simulink model "PROBLEM_2_SUSPENSION_SYSTEM"  (R2020b)
settings: Solver=VariableStepAuto  StartTime=0.0  StopTime=10.0  RelTol=1e-3
model workspace (MAT data in the model file):
  a = [-1.435  -0.2225  -0.0042  -0.0003; 1  0  0  0; 0  1  0  0; 0  0  1  0]
  b = [1; 0; 0; 0]
  c = [0 0 0.0042 0.0003]
  d = 0
  den = [1000 1435 222.5 4.2 0.3]
  num = [4.2 0.3]
  out = Simulink.SimulationOutput
  out.Data.logsout = Simulink.SimulationData.Dataset
  out.Data.logsout.any.Name = 'logsout'
  out.Data.logsout.any.Version = 3
  out.Data.logsout.any.Storage = Simulink.SimulationData.Storage.RamDatasetStorage
  out.Data.logsout.any.Storage.any.Version = 2
  out.Data.logsout.any.Storage.any.Elements{1} = Simulink.SimulationData.Signal
  out.Data.logsout.any.Storage.any.Elements{1}.PortType = 'outport'
  out.Data.logsout.any.Storage.any.Elements{1}.Version = 1
  out.Data.logsout.any.Storage.any.Elements{1}.BlockPath = Simulink.SimulationData.BlockPath
  out.Data.logsout.any.Storage.any.Elements{1}.BlockPath.path = {'PROBLEM_2_SUSPENSION_SYSTEM/Randum Signal Generator'}
  out.Data.logsout.any.Storage.any.Elements{1}.Values = timeseries
  out.Data.logsout.any.Storage.any.Elements{1}.Values.DataInfo = tsdata.datametadata
  out.Data.logsout.any.Storage.any.Elements{1}.Values.DataInfo.Interpolation = tsdata.interpolation
  out.Data.logsout.any.Storage.any.Elements{1}.Values.DataInfo.Interpolation.Fhandle : function handle (value not decoded)
  out.Data.logsout.any.Storage.any.Elements{1}.Values.DataInfo.Interpolation.Name = 'zoh'
  out.Data.logsout.any.Storage.any.Elements{1}.Values.TimeInfo = tsdata.timemetadata
  out.Data.logsout.any.Storage.any.Elements{1}.Values.TimeInfo.Length = 55
  out.Data.logsout.any.Storage.any.Elements{1}.Values.TimeInfo.DuplicateTimes = 0
  out.Data.logsout.any.Storage.any.Elements{1}.Values.TimeInfo.Time_ = [0; 0.000357511978234; 0.0021450718694; 0.0110828713253; 0.0557718686045; 0.255771868605; 0.453364954523; 0.653364954523; 0.853364954523; 1.05336495452; 1.25336495452; 1.45336495452; 1.65336495452; 1.85336495452; 2.05336495452; 2.25336495452; 2.45336495452; 2.65336495452; 2.85336495452; 3.05336495452; 3.25336495452; 3.45336495452; 3.65336495452; 3.85336495452; 4.05336495452; 4.25336495452; 4.45336495452; 4.65336495452; 4.85336495452; 5.05336495452; 5.25336495452; 5.45336495452; 5.65336495452; 5.85336495452; 6.05336495452; 6.25336495452; 6.45336495452; 6.65336495452; 6.85336495452; 7.05336495452; 7.25336495452; 7.45336495452; 7.65336495452; 7.85336495452; 8.05336495452; 8.25336495452; 8.45336495452; 8.65336495452; 8.85336495452; 9.05336495452; 9.25336495452; 9.45336495452; 9.65336495452; 9.85336495452; 10]
  out.Data.logsout.any.Storage.any.Elements{1}.Values.TimeInfo.Initialized = 1
  out.Data.logsout.any.Storage.any.Elements{1}.Values.QualityInfo = tsdata.qualmetadata
  out.Data.logsout.any.Storage.any.Elements{1}.Values.Data_ = [-0.562081627344; -0.905910767571; 0.357729433737; 0.358592811673; 0.869385791882; -0.23299584502; 0.0388327441359; 0.661930692225; -0.930855778945; -0.893076729911; 0.0594003866703; 0.342298768154; -0.984603627578; -0.23316869849; -0.866315524963; -0.165028051084; 0.373545424721; 0.177953285714; 0.860872989456; 0.692333781017; 0.0538575551723; -0.816070218485; 0.307837924598; -0.168001286298; 0.402381188889; 0.820641660979; 0.524396079371; -0.475094012672; -0.905070972585; 0.472163769171; -0.34353154774; 0.265277135775; 0.512820971903; 0.982074771068; -0.269322658549; -0.505922228799; 0.965100572428; 0.445320801551; 0.506711669968; 0.303037149507; -0.854628234103; 0.263269436203; 0.769414257151; -0.454580066472; -0.127177188698; 0.532989555752; -0.0445364699906; -0.524451132642; -0.450186319393; -0.281470041387; -0.666985599169; -0.0269652339755; 0.795312573107; 0.818416203288; -0.878871344905]
  out.Data.logsout.any.Storage.any.Elements{2} = Simulink.SimulationData.Signal
  out.Data.logsout.any.Storage.any.Elements{2}.PortType = 'outport'
  out.Data.logsout.any.Storage.any.Elements{2}.Version = 1
  out.Data.logsout.any.Storage.any.Elements{2}.BlockPath = Simulink.SimulationData.BlockPath
  out.Data.logsout.any.Storage.any.Elements{2}.BlockPath.path = {'PROBLEM_2_SUSPENSION_SYSTEM/transfer Fcn'}
  out.Data.logsout.any.Storage.any.Elements{2}.Values = timeseries
  out.Data.logsout.any.Storage.any.Elements{2}.Values.DataInfo = tsdata.datametadata
  out.Data.logsout.any.Storage.any.Elements{2}.Values.DataInfo.Interpolation = tsdata.interpolation
  out.Data.logsout.any.Storage.any.Elements{2}.Values.DataInfo.Interpolation.Fhandle : function handle (value not decoded)
  out.Data.logsout.any.Storage.any.Elements{2}.Values.DataInfo.Interpolation.Name = 'linear'
  out.Data.logsout.any.Storage.any.Elements{2}.Values.TimeInfo = tsdata.timemetadata
  out.Data.logsout.any.Storage.any.Elements{2}.Values.TimeInfo.Length = 55
  out.Data.logsout.any.Storage.any.Elements{2}.Values.TimeInfo.DuplicateTimes = 0
  out.Data.logsout.any.Storage.any.Elements{2}.Values.TimeInfo.Time_ = [0; 0.000357511978234; 0.0021450718694; 0.0110828713253; 0.0557718686045; 0.255771868605; 0.453364954523; 0.653364954523; 0.853364954523; 1.05336495452; 1.25336495452; 1.45336495452; 1.65336495452; 1.85336495452; 2.05336495452; 2.25336495452; 2.45336495452; 2.65336495452; 2.85336495452; 3.05336495452; 3.25336495452; 3.45336495452; 3.65336495452; 3.85336495452; 4.05336495452; 4.25336495452; 4.45336495452; 4.65336495452; 4.85336495452; 5.05336495452; 5.25336495452; 5.45336495452; 5.65336495452; 5.85336495452; 6.05336495452; 6.25336495452; 6.45336495452; 6.65336495452; 6.85336495452; 7.05336495452; 7.25336495452; 7.45336495452; 7.65336495452; 7.85336495452; 8.05336495452; 8.25336495452; 8.45336495452; 8.65336495452; 8.85336495452; 9.05336495452; 9.25336495452; 9.45336495452; 9.65336495452; 9.85336495452; 10]
  out.Data.logsout.any.Storage.any.Elements{2}.Values.TimeInfo.Initialized = 1
  out.Data.logsout.any.Storage.any.Elements{2}.Values.QualityInfo = tsdata.qualmetadata
  out.Data.logsout.any.Storage.any.Elements{2}.Values.Data_ = [0; -1.79769617365e-14; -5.2545676181e-12; -1.99823284744e-10; 2.68404498816e-08; 6.21540832091e-06; 3.33796218492e-05; 7.66765863418e-05; 0.000135083595736; 0.000213011794581; 0.000285578520613; 0.000332316235162; 0.000358070547876; 0.000369568723865; 0.000351228771915; 0.000296660223416; 0.000195857608614; 5.50687074212e-05; -0.000108048435281; -0.000277752458139; -0.000430433823258; -0.000551722669519; -0.000648653887148; -0.000740766542261; -0.000827409016616; -0.000909310861356; -0.000975860507589; -0.00100979959918; -0.00100725901542; -0.000988637627288; -0.000975312475436; -0.000962789878736; -0.000954142409177; -0.000942195435816; -0.000911411736333; -0.000846273078161; -0.000758722946634; -0.000660598580283; -0.000535940247566; -0.000375849169482; -0.000175939543201; 5.71877376748e-05; 0.000300614028672; 0.000556114151792; 0.000833607921404; 0.00112060861772; 0.00141185503937; 0.00171473594978; 0.00202402370516; 0.00232406756258; 0.00260314669473; 0.00285406285464; 0.00306803595231; 0.00325363092994; 0.00338660884517]
  out.Data.tout = [0; 0.000357511978234; 0.0021450718694; 0.0110828713253; 0.0557718686045; 0.255771868605; 0.453364954523; 0.653364954523; 0.853364954523; 1.05336495452; 1.25336495452; 1.45336495452; 1.65336495452; 1.85336495452; 2.05336495452; 2.25336495452; 2.45336495452; 2.65336495452; 2.85336495452; 3.05336495452; 3.25336495452; 3.45336495452; 3.65336495452; 3.85336495452; 4.05336495452; 4.25336495452; 4.45336495452; 4.65336495452; 4.85336495452; 5.05336495452; 5.25336495452; 5.45336495452; 5.65336495452; 5.85336495452; 6.05336495452; 6.25336495452; 6.45336495452; 6.65336495452; 6.85336495452; 7.05336495452; 7.25336495452; 7.45336495452; 7.65336495452; 7.85336495452; 8.05336495452; 8.25336495452; 8.45336495452; 8.65336495452; 8.85336495452; 9.05336495452; 9.25336495452; 9.45336495452; 9.65336495452; 9.85336495452; 10]
  out.Metadata = Simulink.SimulationMetadata
  out.Metadata.ModelInfo.ModelName = 'PROBLEM_2_SUSPENSION_SYSTEM'
  out.Metadata.ModelInfo.ModelVersion = '1.3'
  out.Metadata.ModelInfo.ModelFilePath = 'D:\KPIT\PROBLEM_2\Simulink Model\PROBLEM_2_SUSPENSION_SYSTEM.slx'
  out.Metadata.ModelInfo.UserID = 'intel'
  out.Metadata.ModelInfo.MachineName = 'DESKTOP-HTPAP2M'
  out.Metadata.ModelInfo.Platform = 'PCWIN64'
  out.Metadata.ModelInfo.ModelStructuralChecksum = [2786829521; 1170271611; 2990410611; 2656339131]
  out.Metadata.ModelInfo.SimulationMode = 'normal'
  out.Metadata.ModelInfo.StartTime = 0
  out.Metadata.ModelInfo.StopTime = 10
  out.Metadata.ModelInfo.SolverInfo.Type = 'Variable-Step'
  out.Metadata.ModelInfo.SolverInfo.Solver = 'ode45'
  out.Metadata.ModelInfo.SolverInfo.MaxStepSize = 0.2
  out.Metadata.ModelInfo.SimulinkVersion.Name = 'Simulink'
  out.Metadata.ModelInfo.SimulinkVersion.Version = '10.2'
  out.Metadata.ModelInfo.SimulinkVersion.Release = '(R2020b)'
  out.Metadata.ModelInfo.SimulinkVersion.Date = '29-Jul-2020'
  out.Metadata.ModelInfo.LoggingInfo.LoggingToFile = 'off'
  out.Metadata.TimingInfo.WallClockTimestampStart = '2020-12-04 22:57:30'
  out.Metadata.TimingInfo.WallClockTimestampStop = '2020-12-04 22:57:32'
  out.Metadata.TimingInfo.InitializationElapsedWallTime = 1.1649333
  out.Metadata.TimingInfo.ExecutionElapsedWallTime = 0.3698049
  out.Metadata.TimingInfo.TerminationElapsedWallTime = 0.268201
  out.Metadata.TimingInfo.TotalElapsedWallTime = 1.8029392
  out.Metadata.TimingInfo.ProfilerData = 'Profiler is not enabled'
  out.Metadata.ExecutionInfo.StopEvent = 'ReachedStopTime'
  out.Metadata.ExecutionInfo.StopEventSource = []
  out.Metadata.ExecutionInfo.StopEventDescription = 'Reached stop time of 10'
  out.Metadata.ExecutionInfo.ErrorDiagnostic = []
  out.Metadata.ExecutionInfo.WarningDiagnostics.Diagnostic = MSLDiagnostic
  out.Metadata.ExecutionInfo.WarningDiagnostics.Diagnostic.identifier = 'Simulink:blocks:SiggenRandomWaveObsolete'
  out.Metadata.ExecutionInfo.WarningDiagnostics.Diagnostic.message = 'The "random" waveform selection of ''<a href="matlab:open_and_hilite_hyperlink (''PROBLEM_2_SUSPENSION_SYSTEM/Randum Signal Generator'',''error'')">PROBLEM_2_SUSPENSION_SYSTEM/Randum Signal Generator</a>'' is provided for backwards compatibility. It will be removed in a future version and should be replaced with the appropriate random number generator'
  out.Metadata.ExecutionInfo.WarningDiagnostics.Diagnostic.paths = {'PROBLEM_2_SUSPENSION_SYSTEM/Randum Signal Generator'}
  out.Metadata.ExecutionInfo.WarningDiagnostics.Diagnostic.arguments = {'PROBLEM_2_SUSPENSION_SYSTEM/Randum Signal Generator'}
  out.Metadata.ExecutionInfo.WarningDiagnostics.Diagnostic.stack = struct([])
  out.Metadata.ExecutionInfo.WarningDiagnostics.SimulationPhase = 'Initialization'
  out.Metadata.ExecutionInfo.WarningDiagnostics.SimulationTime = []
  out.Metadata.AppInfo = struct()
settings Model: OrderedModelArguments=off  Creator=intel  LastModifiedBy=intel

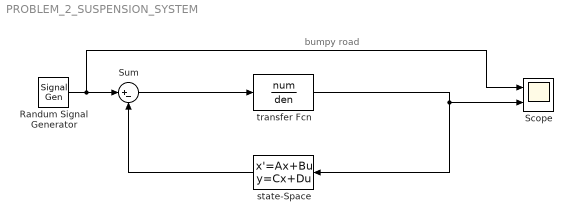
== system PROBLEM_2_SUSPENSION_SYSTEM ==
  note: bumpy road
  Randum Signal Generator : SignalGenerator  WaveForm=random  Units=rad/sec
  Scope : Scope  NumInputPorts=2
  Sum : Sum  Inputs=|+-
  state-Space : StateSpace  A=a  B=b  C=c  D=d  InitialCondition=0
  transfer Fcn : TransferFcn  Numerator=num  Denominator=den
  wires:
  Sum/1 -> transfer Fcn/1
  transfer Fcn/1 -> Scope/2, state-Space/1
  Randum Signal Generator/1 -> Scope/1, Sum/1
  state-Space/1 -> Sum/2
